simulink model "lab5_221147"  (R2022b)
settings: Solver=VariableStepAuto  StartTime=0.0  StopTime=10.0  RelTol=1e-3
values from neighbouring files (symbols this model uses):
  Kc = 9.9*0.026    (= 0.2574)    [lab6.m]
  tau_i = 9.9    [lab6.m]
settings Model: Creator=Administrator  LastModifiedBy=Administrator

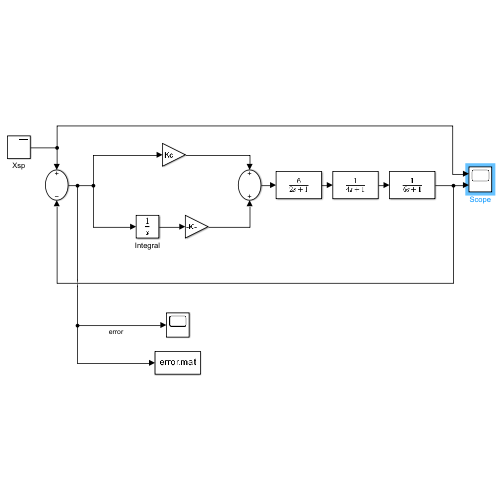
[thumbnail: Simulink's stored preview of the top-level diagram]
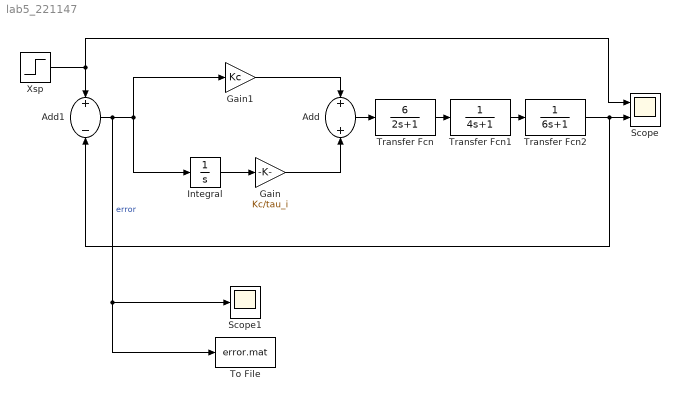
== system lab5_221147 ==
  Add : Sum
  Add1 : Sum  Inputs=+-
  Gain : Gain  Gain=Kc/tau_i
  Gain1 : Gain  Gain=Kc
  Integral : Integrator
  Scope : Scope  NumInputPorts=2
  Scope1 : Scope
  To File : ToFile  Filename=error.mat  MatrixName=e  SampleTime=0.1
  Transfer Fcn : TransferFcn  Numerator=[6]  Denominator=[2 1]
  Transfer Fcn1 : TransferFcn  Denominator=[4 1]
  Transfer Fcn2 : TransferFcn  Denominator=[6 1]
  Xsp : Step  Time=0  SampleTime=0.1
  wires:
  Integral/1 -> Gain/1
  Gain/1 -> Add/2
  Gain1/1 -> Add/1
  Transfer Fcn/1 -> Transfer Fcn1/1
  Transfer Fcn1/1 -> Transfer Fcn2/1
  Add/1 -> Transfer Fcn/1
  Xsp/1 -> Add1/1, Scope/1
  Transfer Fcn2/1 -> Add1/2, Scope/2
  Add1/1 -> To File/1, Scope1/1, Gain1/1, Integral/1  "error"
